simulink model "LeftCameraAgent"  (Simulink 6.2)
settings: Solver=ode45  StartTime=0.0  StopTime=10.0  RelTol=1e-3
settings Model: LastModifiedBy=suarezjl
settings DataIOCC: SignalLoggingName=sigsOut
settings HardwareCC: TargetUnknown=on

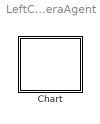
== system LeftCameraAgent ==
  Chart : Stateflow chart

== stateflow chart Chart ==
  state Initial
    \\Sally\CogDemo\LeftCameraAgent\FrameGrabber.Initialize()
    \\Sally\CogDemo\LeftCameraAgent\FrameGrabber.ObtainImage()
    \\Sally\CogDemo\LeftCameraAgent\FrameGrabber.ObtainImage()
    \\Sally\CogDemo\LeftCameraAgent\ColorBarney.Initial()
    \\Sally\CogDemo\LeftCameraAgent\ColorBarney.LoadColorModel()
  state Segmentation
    \\Sally\CogDemo\LeftCameraAgent\FrameGrabber.ObtainImage()
    \\Sally\CogDemo\LeftCameraAgent\ColorSegmenter.DoSegment()
  (default) -> Initial : Start
  Initial -> Segmentation : Always
  Segmentation -> Segmentation : Always
